simulink model "model2"  (R2014b)
settings: Solver=ode45  StartTime=0.0  StopTime=90  RelTol=1e-3
settings Model: Creator=Shane Reynolds  LastModifiedBy=Shane Reynolds

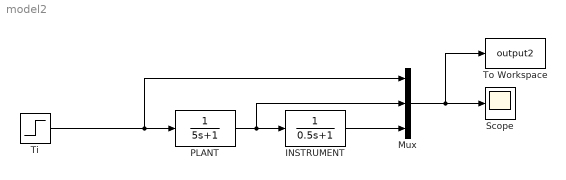
== system model2 ==
  INSTRUMENT : TransferFcn  Denominator=[0.5 1]
  Mux : Mux  Inputs=3
  PLANT : TransferFcn  Denominator=[5 1]
  Scope : Scope
  Ti : Step  After=10  SampleTime=0
  To Workspace : ToWorkspace  VariableName=output2  SaveFormat=Timeseries  SampleTime=-1
  wires:
  PLANT/1 -> Mux/2, INSTRUMENT/1
  Ti/1 -> Mux/1, PLANT/1
  INSTRUMENT/1 -> Mux/3
  Mux/1 -> To Workspace/1, Scope/1
